simulink model "single_joint_controller_struct"  (R2023b)
settings: Solver=FixedStepDiscrete  StartTime=0.0  StopTime=1.0  FixedStep=0.001  RelTol=1e-3
settings Model: Creator=user  LastModifiedBy=user
settings DebuggingCC: BusObjectLabelMismatch=error
settings HardwareCC: ProdBitPerLong=64  ProdHWDeviceType=Intel->x86-64 (Linux 64)  TargetBitPerLong=64  TargetBitPerPointer=64  TargetBitPerSizeT=64  TargetBitPerPtrDiffT=64  TargetLargestAtomicFloat=Float  TargetIntDivRoundTo=Zero  TargetEndianess=LittleEndian  TargetWordSize=64  TargetHWDeviceType=Intel->x86-64 (Linux 64)  ProdEqTarget=off
settings RTWCC: GenerateReport=on

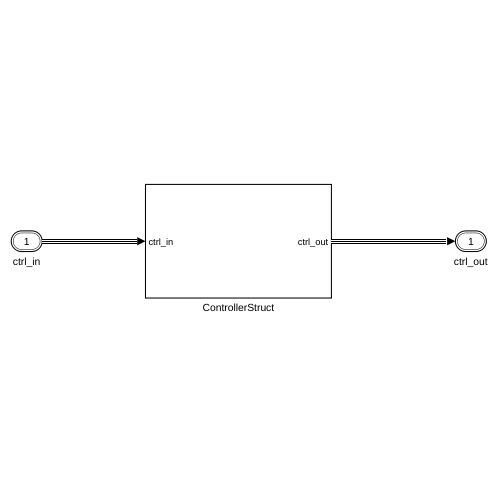
[thumbnail: Simulink's stored preview of the top-level diagram]
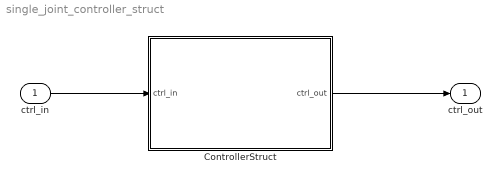
== system single_joint_controller_struct ==
  ctrl_in : Inport  OutDataTypeStr=Bus: ControllerInputBus
  ControllerStruct : Subsystem  RTWFcnName=usr_pid  RTWFileName=usr_pid
      settings: RTWFcnNameOpts=User specified  RTWFileNameOpts=User specified
  ctrl_out : Outport  OutDataTypeStr=Bus: ControllerOutputBus
  wires:
  ctrl_in/1 -> ControllerStruct/1(ctrl_in)
  ControllerStruct/1(ctrl_out) -> ctrl_out/1

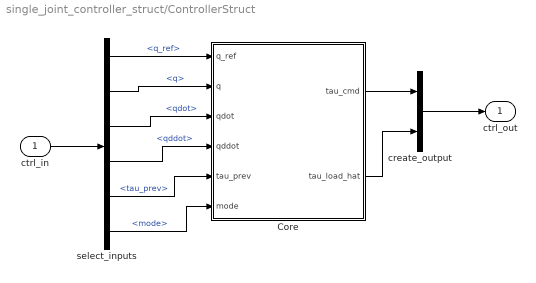
== system single_joint_controller_struct/ControllerStruct ==
  ctrl_in : Inport  OutDataTypeStr=Bus: ControllerInputBus
  Core : MATLAB Function  TreatAsAtomicUnit=on
  create_output : BusCreator  Inputs=2  OutDataTypeStr=Bus: ControllerOutputBus
  select_inputs : BusSelector  OutputSignals=q_ref,q,qdot,qddot,tau_prev,mode
  ctrl_out : Outport  OutDataTypeStr=Bus: ControllerOutputBus
  wires:
  Core/2(tau_load_hat) -> create_output/2
  Core/1(tau_cmd) -> create_output/1
  create_output/1 -> ctrl_out/1
  select_inputs/6 -> Core/6(mode)  "<mode>"
  select_inputs/4 -> Core/4(qddot)  "<qddot>"
  select_inputs/5 -> Core/5(tau_prev)  "<tau_prev>"
  select_inputs/3 -> Core/3(qdot)  "<qdot>"
  select_inputs/2 -> Core/2(q)  "<q>"
  select_inputs/1 -> Core/1(q_ref)  "<q_ref>"
  ctrl_in/1 -> select_inputs/1

== matlab function single_joint_controller_struct/ControllerStruct/Core ==
  data: q_ref input; tau_cmd output; q input; qdot input; qddot input; tau_prev input; mode input; tau_load_hat output
function [tau_cmd, tau_load_hat] = fcn(q_ref, q, qdot, qddot, tau_prev, mode)
%#codegen
persistent integral_e dob_hat
if isempty(integral_e)
    integral_e = fi(0, 1, 16, 13);
    dob_hat = fi(0, 1, 16, 13);
end
q_ref_f = fi(q_ref, 1, 16, 12);
q_f = fi(q, 1, 16, 12);
qdot_f = fi(qdot, 1, 16, 8);
qddot_f = fi(qddot, 1, 16, 4);
tau_prev_f = fi(tau_prev, 1, 16, 12);
mode_f = mode;
Ts = fi(0.001, 1, 16, 15);
tau_limit = fi(1.5, 1, 16, 13);
integral_limit = fi(0.40000000000000002, 1, 16, 13);
tau_hat_limit = fi(0.80000000000000004, 1, 16, 13);
Kp_pid = fi(8, 1, 16, 10);
Ki_pid = fi(6, 1, 16, 10);
Kd_pid = fi(0.45000000000000001, 1, 16, 14);
Kp_dob = fi(8, 1, 16, 10);
Kd_dob = fi(0.45000000000000001, 1, 16, 14);
Jn_dob = fi(0.01, 1, 16, 15);
bn_dob = fi(0.02, 1, 16, 15);
alpha_dob = fi(0.19741016454517191, 1, 16, 14);
K_imp = fi(4, 1, 16, 10);
D_imp = fi(0.38, 1, 16, 14);
e = fi(q_ref_f - q_f, 1, 16, 12);
tau_cmd = fi(0, 1, 16, 13);
tau_load_hat = fi(0, 1, 16, 13);
if mode_f < uint8(2)
    integral_e = fi(integral_e + Ts*e, 1, 16, 13);
    if integral_e > integral_limit
        integral_e = integral_limit;
    elseif integral_e < -integral_limit
        integral_e = -integral_limit;
    end
    tau_cmd = fi(Kp_pid*e + Ki_pid*integral_e - Kd_pid*qdot_f, 1, 16, 13);
elseif mode_f < uint8(3)
    raw_load = fi(tau_prev_f - Jn_dob*qddot_f - bn_dob*qdot_f, 1, 16, 13);
    dob_hat = fi(dob_hat + alpha_dob*(raw_load - dob_hat), 1, 16, 13);
    if dob_hat > tau_hat_limit
        dob_hat = tau_hat_limit;
    elseif dob_hat < -tau_hat_limit
        dob_hat = -tau_hat_limit;
    end
    tau_load_hat = dob_hat;
    tau_cmd = fi(Kp_dob*e - Kd_dob*qdot_f + tau_load_hat, 1, 16, 13);
else
    tau_cmd = fi(K_imp*e - D_imp*qdot_f, 1, 16, 13);
end
if tau_cmd > tau_limit
    tau_cmd = tau_limit;
elseif tau_cmd < -tau_limit
    tau_cmd = -tau_limit;
end
end
